simulink model "mavsim_test"  (R2021b)
settings: Solver=ode45  StartTime=0.0  StopTime=25  RelTol=1e-3  EnableMultiTasking=on
InitFcn:
  | main2;
values from neighbouring files (symbols this model uses):
  K_lat = [-0.304148873535 -1.33998556637 -1.58184554862 -3.24340069218 -0.0524623541154 0.634644996647 0.505860523594 -0.0512969698311 2.73325585285 -4.90568206591 -2.64587570986 1.90053400734 ... (16 elements, 2x8)]    [Lat.mat]
  K_lon = [4.2230540418 -9.87666863045 3.92050270009 -1.00690047299 2.23086857596 8.41143486725 1.21871720558 2.14878438432 33.3955354841 -15.8285944163 -6.80667379316 15.8766469128 ... (16 elements, 2x8)]    [Lon.mat]
  P =     [P.mat]    (also in expand_path_points.m = P1 *(1 - t) + t * P2)
undefined symbols (not defined in the file or in its folder): forces_moments
settings Model: Creator=beard  LastModifiedBy=hpShe
settings SolverCC: AlgebraicLoopSolver=TrustRegion
settings DataIOCC: ExternalInput=[]  InitialState=[]  LimitDataPoints=on  LoadExternalInput=on  LoadInitialState=on  SaveFormat=Array  SignalLoggingSaveFormat=ModelDataLogs  ReturnWorkspaceOutputs=off
settings OptimizationCC: DefaultParameterBehavior=Inlined  BufferReuse=off  ExpressionDepthLimit=2147483647  InitFltsAndDblsToZero=on  LifeSpan=inf
settings DebuggingCC: UnderspecifiedInitializationDetection=Classic  MergeDetectMultiDrivingBlocksExec=none  SolverPrmCheckMsg=warning  FcnCallInpInsideContextMsg=warning  StateNameClashWarn=warning  InitInArrayFormatMsg=none  SFUnexpectedBacktrackingDiag=warning  SFNoUnconditionalDefaultTransitionDiag=warning  SFExecutionAtInitializationDiag=none  SFMachineParentedDataDiag=warning  ArithmeticOperatorsInVariantConditions=warning
settings HardwareCC: ProdBitPerPointer=32  ProdBitPerSizeT=32  ProdBitPerPtrDiffT=32  ProdLargestAtomicFloat=None  ProdIntDivRoundTo=Undefined  ProdEndianess=Unspecified  ProdWordSize=32  ProdHWDeviceType=32-bit Generic
settings ModelReferenceCC: PropagateSignalLabelsOutOfModel=off
settings SFSimCC: SimUseLocalCustomCode=off  CustomCodeUndefinedFunction=UseInterfaceOnly
settings RTWCC: RTWUseLocalCustomCode=off
settings CodeAppCC: StateflowObjectComments=on
settings GRTTargetCC: TargetLangStandard=C89/C90 (ANSI)  CombineOutputUpdateFcns=off  GRTInterface=on
settings ConfigComp: CovMetricSettings=dw  CovSaveCumulativeToWorkspaceVar=on  CovSaveSingleToWorkspaceVar=on  CovExternalEMLEnable=off

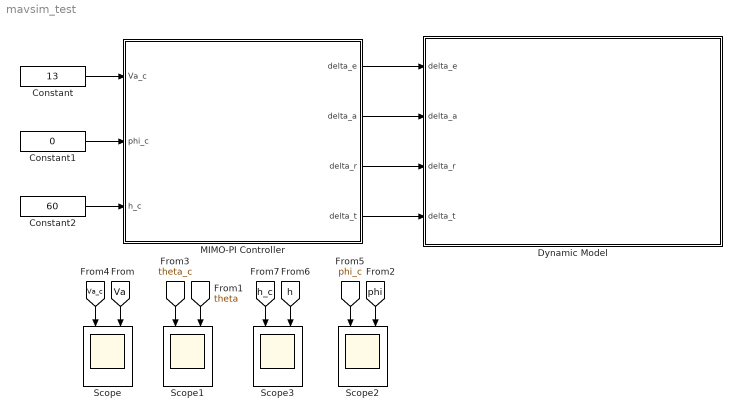
== system mavsim_test ==
  Constant : Constant  Value=13
  Constant1 : Constant  Value=0
  Constant2 : Constant  Value=60
  "Dynamic Model " : Subsystem
  MIMO-PI Controller : Subsystem
  Scope{,1..3} (4 alike) : Scope  NumInputPorts=2
  wires:
  Constant/1 -> MIMO-PI Controller/1(Va_c)
  [Va] -> Scope/2
  [theta] -> Scope1/2
  [phi] -> Scope2/2
  MIMO-PI Controller/1(delta_e) -> "Dynamic Model "/1(delta_e)
  MIMO-PI Controller/2(delta_a) -> "Dynamic Model "/2(delta_a)
  MIMO-PI Controller/3(delta_r) -> "Dynamic Model "/3(delta_r)
  MIMO-PI Controller/4(delta_t) -> "Dynamic Model "/4(delta_t)
  [theta_c] -> Scope1/1
  [Va_c] -> Scope/1
  [phi_c] -> Scope2/1
  Constant1/1 -> MIMO-PI Controller/2(phi_c)
  Constant2/1 -> MIMO-PI Controller/3(h_c)
  [h_c] -> Scope3/1
  [h] -> Scope3/2

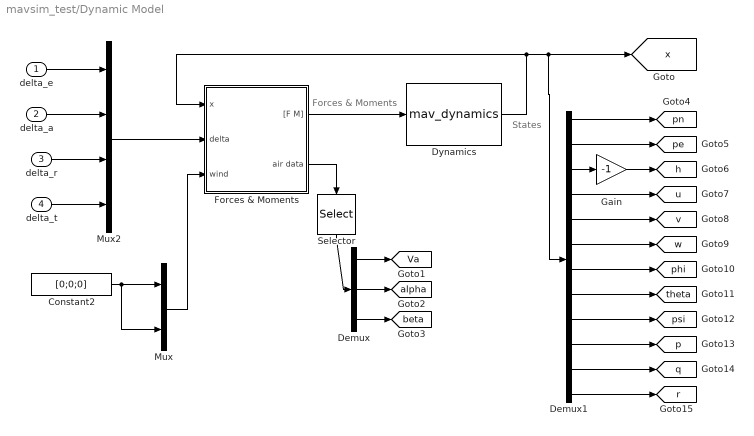
== system mavsim_test/Dynamic Model  ==
  note: Forces & Moments
  note: States
  delta_e : Inport
  delta_a : Inport  Port=2
  delta_r : Inport  Port=3
  delta_t : Inport  Port=4
  Constant2 : Constant  Value=[0;0;0]
  Demux : Demux  Outputs=3
  Demux1 : Demux  Outputs=12
  Dynamics : S-Function  FunctionName=mav_dynamics  Parameters=mass,Jx,Jy,Jz,Jxz,pn0,pe0,pd0,u0,v0,w0,phi0,theta0,psi0,p0,q0,r0  SFunctionDeploymentMode=off  EnableBusSupport=off  mask{mass=P.mass, Jx=P.Jx, Jy=P.Jy, Jz=P.Jz, Jxz=P.Jxz, pn0=P.pn0, pe0=P.pe0, pd0=P.pd0, u0=P.u0, v0=P.v0, w0=P.w0, phi0=P.phi0, theta0=P.theta0, psi0=P.psi0, p0=P.p0, q0=P.q0, r0=P.r0}
      mask prompts: pn0 "Initial North position"; pe0 "Initial East position"; pd0 "Initial Down position"; u0 "Initial velocy u0"; v0 "Initial velocity v0"; w0 "Initial velocity w0"; phi0 "Initial roll angle"; theta0 "Initial pitch angle"; psi0 "Initial yaw angle"; p0 "Initial roll rate"; q0 "Initial pitch rate"; r0 "Initial yaw rate"
  Forces & Moments : Subsystem
  Gain : Gain  Gain=-1
  Mux : Mux  Inputs=2
  Mux2 : Mux
  Selector : Selector  InputPortWidth=6  IndexOptions=Index vector (dialog)  Indices=[1 2 3]  OutputSizes=1
  tag scope: Va=global, alpha=global, beta=global, h=global, p=global, pe=global, phi=global, pn=global, psi=global, q=global, r=global, theta=global, u=global, v=global, w=global, x=global
  wires:
  delta_e/1 -> Mux2/1
  Constant2/1 -> Mux/1, Mux/2
  Mux2/1 -> Forces & Moments/2(delta)
  Mux/1 -> Forces & Moments/3(wind)
  delta_r/1 -> Mux2/3
  Forces & Moments/1("[F M]") -> Dynamics/1
  delta_t/1 -> Mux2/4
  delta_a/1 -> Mux2/2
  Dynamics/1 -> Demux1/1, [x], Forces & Moments/1(x)
  Forces & Moments/2(air data) -> Selector/1
  Demux/3 -> [beta]
  Demux/1 -> [Va]
  Demux/2 -> [alpha]
  Selector/1 -> Demux/1
  Demux1/1 -> [pn]
  Demux1/2 -> [pe]
  Demux1/3 -> Gain/1
  Gain/1 -> [h]
  Demux1/4 -> [u]
  Demux1/5 -> [v]
  Demux1/6 -> [w]
  Demux1/7 -> [phi]
  Demux1/8 -> [theta]
  Demux1/9 -> [psi]
  Demux1/10 -> [p]
  Demux1/11 -> [q]
  Demux1/12 -> [r]

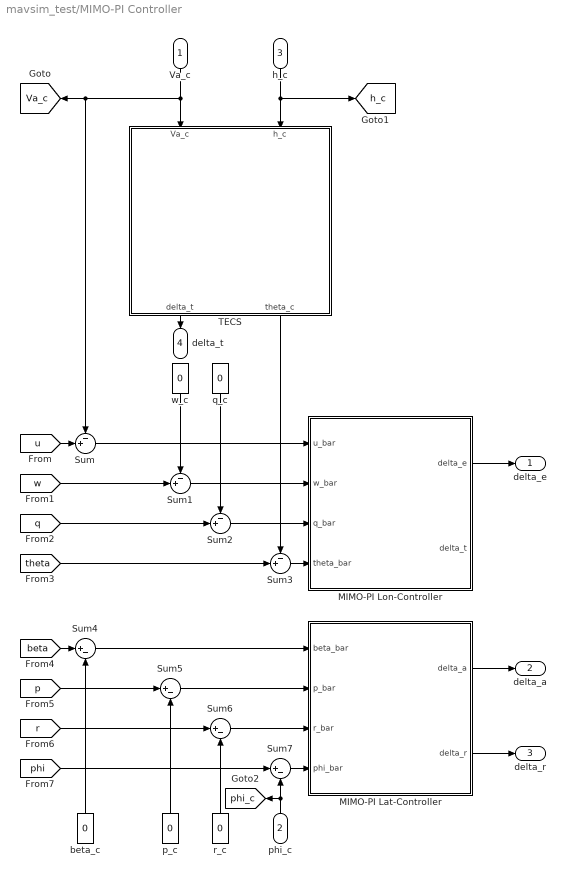
== system mavsim_test/MIMO-PI Controller ==
  Va_c : Inport
  phi_c : Inport  Port=2
  h_c : Inport  Port=3
  MIMO-PI Lat-Controller : Subsystem
  MIMO-PI Lon-Controller : Subsystem
  Sum{,1..3} (4 alike) : Sum  Inputs=-+|
  Sum{4..7} (4 alike) : Sum  Inputs=|+-
  TECS : Subsystem
  beta_c : Constant  Value=0
  p_c : Constant  Value=0
  q_c : Constant  Value=0
  r_c : Constant  Value=0
  w_c : Constant  Value=0
  delta_e : Outport
  delta_a : Outport  Port=2
  delta_r : Outport  Port=3
  delta_t : Outport  Port=4
  tag scope: Va_c=global, h_c=global, phi_c=global
  wires:
  MIMO-PI Lat-Controller/2(delta_r) -> delta_r/1
  Sum4/1 -> MIMO-PI Lat-Controller/1(beta_bar)
  Sum7/1 -> MIMO-PI Lat-Controller/4(phi_bar)
  MIMO-PI Lon-Controller/1(delta_e) -> delta_e/1
  [w] -> Sum1/2
  Sum/1 -> MIMO-PI Lon-Controller/1(u_bar)
  [q] -> Sum2/2
  MIMO-PI Lat-Controller/1(delta_a) -> delta_a/1
  phi_c/1 -> [phi_c], Sum7/2
  r_c/1 -> Sum6/2
  [p] -> Sum5/1
  Sum2/1 -> MIMO-PI Lon-Controller/3(q_bar)
  [beta] -> Sum4/1
  [u] -> Sum/2
  q_c/1 -> Sum2/1
  [theta] -> Sum3/2
  Sum1/1 -> MIMO-PI Lon-Controller/2(w_bar)
  Sum6/1 -> MIMO-PI Lat-Controller/3(r_bar)
  Va_c/1 -> TECS/1(Va_c), Sum/1, [Va_c]
  Sum5/1 -> MIMO-PI Lat-Controller/2(p_bar)
  Sum3/1 -> MIMO-PI Lon-Controller/4(theta_bar)
  w_c/1 -> Sum1/1
  p_c/1 -> Sum5/2
  [phi] -> Sum7/1
  beta_c/1 -> Sum4/2
  [r] -> Sum6/1
  TECS/2(theta_c) -> Sum3/1
  TECS/1(delta_t) -> delta_t/1
  h_c/1 -> [h_c], TECS/2(h_c)

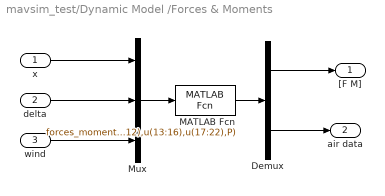
== system mavsim_test/Dynamic Model /Forces & Moments ==
  x : Inport
  delta : Inport  Port=2
  wind : Inport  Port=3
  Demux : Demux  Outputs=[6;6]
  MATLAB Fcn : MATLABFcn  MATLABFcn=forces_moments(u(1:12),u(13:16),u(17:22),P)  OutputDimensions=12
  Mux : Mux  Inputs=3
  "[F M]" : Outport
  air data : Outport  Port=2
  wires:
  x/1 -> Mux/1
  delta/1 -> Mux/2
  wind/1 -> Mux/3
  MATLAB Fcn/1 -> Demux/1
  Demux/1 -> "[F M]"/1
  Mux/1 -> MATLAB Fcn/1
  Demux/2 -> air data/1

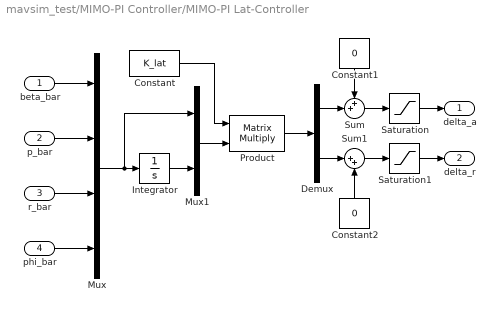
== system mavsim_test/MIMO-PI Controller/MIMO-PI Lat-Controller ==
  beta_bar : Inport
  p_bar : Inport  Port=2
  r_bar : Inport  Port=3
  phi_bar : Inport  Port=4
  Constant : Constant  Value=K_lat
  Constant1 : Constant  Value=0
  Constant2 : Constant  Value=0
  Demux : Demux  Outputs=2
  Integrator : Integrator
  Mux : Mux
  Mux1 : Mux  Inputs=2
  Product : Product  Multiplication=Matrix(*)
  Saturation : Saturate  UpperLimit=pi/4  LowerLimit=-pi/4
  Saturation1 : Saturate  UpperLimit=pi/4  LowerLimit=-pi/4
  Sum : Sum  Inputs=++|
  Sum1 : Sum  Inputs=|++
  delta_a : Outport
  delta_r : Outport  Port=2
  wires:
  phi_bar/1 -> Mux/4
  r_bar/1 -> Mux/3
  p_bar/1 -> Mux/2
  beta_bar/1 -> Mux/1
  Mux/1 -> Mux1/1, Integrator/1
  Product/1 -> Demux/1
  Integrator/1 -> Mux1/2
  Mux1/1 -> Product/2
  Constant/1 -> Product/1
  Saturation/1 -> delta_a/1
  Saturation1/1 -> delta_r/1
  Demux/1 -> Sum/2
  Sum/1 -> Saturation/1
  Demux/2 -> Sum1/1
  Sum1/1 -> Saturation1/1
  Constant1/1 -> Sum/1
  Constant2/1 -> Sum1/2

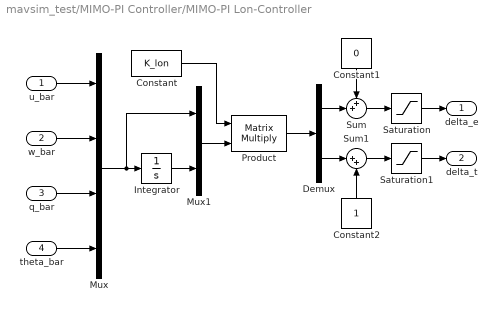
== system mavsim_test/MIMO-PI Controller/MIMO-PI Lon-Controller ==
  u_bar : Inport
  w_bar : Inport  Port=2
  q_bar : Inport  Port=3
  theta_bar : Inport  Port=4
  Constant : Constant  Value=K_lon
  Constant1 : Constant  Value=0
  Constant2 : Constant
  Demux : Demux  Outputs=2
  Integrator : Integrator
  Mux : Mux
  Mux1 : Mux  Inputs=2
  Product : Product  Multiplication=Matrix(*)
  Saturation : Saturate  UpperLimit=pi/4  LowerLimit=-pi/4
  Saturation1 : Saturate  UpperLimit=1  LowerLimit=0
  Sum : Sum  Inputs=++|
  Sum1 : Sum  Inputs=|++
  delta_e : Outport
  delta_t : Outport  Port=2
  wires:
  theta_bar/1 -> Mux/4
  q_bar/1 -> Mux/3
  w_bar/1 -> Mux/2
  u_bar/1 -> Mux/1
  Mux/1 -> Mux1/1, Integrator/1
  Product/1 -> Demux/1
  Integrator/1 -> Mux1/2
  Mux1/1 -> Product/2
  Constant/1 -> Product/1
  Saturation/1 -> delta_e/1
  Saturation1/1 -> delta_t/1
  Demux/1 -> Sum/2
  Sum/1 -> Saturation/1
  Demux/2 -> Sum1/1
  Sum1/1 -> Saturation1/1
  Constant1/1 -> Sum/1
  Constant2/1 -> Sum1/2

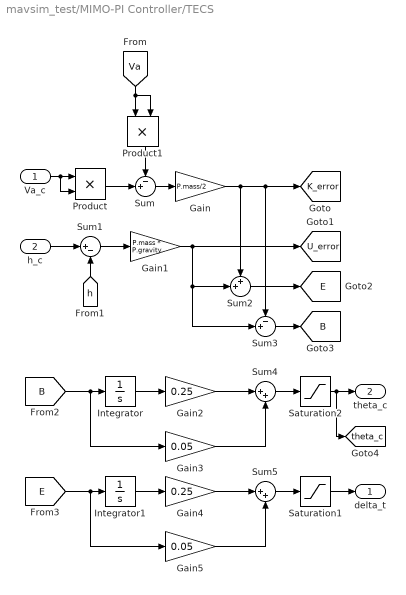
== system mavsim_test/MIMO-PI Controller/TECS ==
  Va_c : Inport
  h_c : Inport  Port=2
  Gain : Gain  Gain=P.mass/2
  Gain1 : Gain  Gain=P.mass * P.gravity
  Gain2 : Gain  Gain=0.25
  Gain3 : Gain  Gain=0.05
  Gain4 : Gain  Gain=0.25
  Gain5 : Gain  Gain=0.05
  Integrator : Integrator
  Integrator1 : Integrator
  Product : Product
  Product1 : Product
  Saturation1 : Saturate  UpperLimit=1  LowerLimit=0
  Saturation2 : Saturate  UpperLimit=pi/4  LowerLimit=-pi/6
  Sum : Sum  Inputs=-+|
  Sum1 : Sum  Inputs=|+-
  Sum2 : Sum  Inputs=++|
  Sum3 : Sum  Inputs=-+|
  Sum4 : Sum  Inputs=|++
  Sum5 : Sum  Inputs=|++
  delta_t : Outport
  theta_c : Outport  Port=2
  tag scope: B=global, E=global, K_error=global, U_error=global, theta_c=global
  wires:
  Va_c/1 -> Product/2, Product/1
  Product/1 -> Sum/2
  [Va] -> Product1/2, Product1/1
  Product1/1 -> Sum/1
  Sum/1 -> Gain/1
  Gain/1 -> [K_error], Sum3/1, Sum2/1
  h_c/1 -> Sum1/1
  [h] -> Sum1/2
  Sum1/1 -> Gain1/1
  Gain1/1 -> [U_error], Sum2/2, Sum3/2
  Sum2/1 -> [E]
  Sum3/1 -> [B]
  Sum5/1 -> Saturation1/1
  Saturation1/1 -> delta_t/1
  [B] -> Gain3/1, Integrator/1
  Integrator/1 -> Gain2/1
  Gain2/1 -> Sum4/1
  Gain3/1 -> Sum4/2
  [E] -> Gain5/1, Integrator1/1
  Integrator1/1 -> Gain4/1
  Gain4/1 -> Sum5/1
  Gain5/1 -> Sum5/2
  Sum4/1 -> Saturation2/1
  Saturation2/1 -> [theta_c], theta_c/1
